simulink model "Emergency_Power_R2020a"  (R2020a)
settings: Solver=VariableStepAuto  StartTime=0.0  StopTime=10.0  RelTol=1e-3
undefined symbols (not defined in the file or in its folder): Ion, Lithium
libraries: electricdrivelib x29, powerlib x13
settings Model: Creator=YXL1108  LastModifiedBy=YXL1108

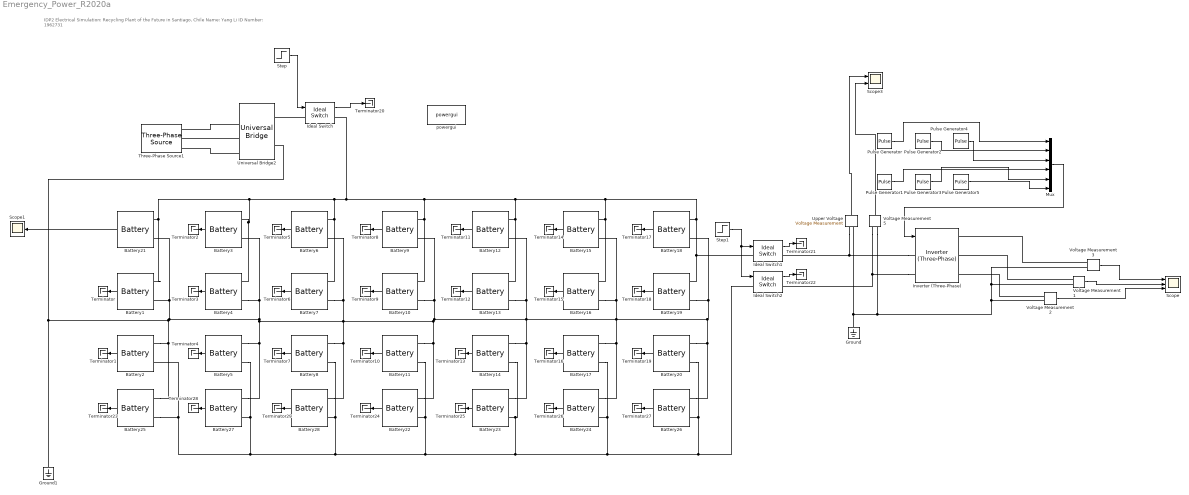
== system Emergency_Power_R2020a ==
  note: IDP2 Electrical Simulation: Recycling Plant of the Future in Santiago, Chile
      | Name: Yang Li
      | ID Number: 1962731
  Battery{1..28} (28 alike) : electricdrivelib/Extra Sources/Battery  BatType=Lithium-Ion  ShowTempParam=off  ThermalPreset=no  ShowAgeParam=off  NomV=Battery_nominal_v  NomQ=Rated_capacity  SOC=100  Batt_Tr=30  PresetModel=on  MaxQ=1000000  MinV=285  FullV=442.3151  Dis_rate=434782.6087  R=3.8e-06  Normal_OP=904347.8261  expZone="[410.546624      49130.4348]"  current=[6.5 13 32.5]  Units=Time  Tci=20  NomT=20  T2=-30  MaxQ2=4.8  FullV2=7.1  Normal_OP2=5.655  expZone2="[6.58           1]"  Rca=0.6  ti=2000  Dp=0  Neq0=0  Tsim=1e6  Ta1=25  Qeol=5.4*0.9  Reol=0.013333*1.2  Char_age=[2.3478, 3]  Dis_age=[2.3478, 10]  N1=1500  N2=10500  N3=1000  N4=1400  Ta2=45  N5=950
  Ground : powerlib/Elements/Ground  LConnTagsString=a
  Ground1 : powerlib/Elements/Ground  LConnTagsString=a
  Ideal Switch : powerlib/Power Electronics/Ideal Switch  Ron=0.001  Lon=0  IC=0  Rs=1e-5  Cs=inf  Measurements=on
  Ideal Switch1 : powerlib/Power Electronics/Ideal Switch  Ron=0.001  Lon=0  IC=0  Rs=1e-5  Cs=inf  Measurements=on
  Ideal Switch2 : powerlib/Power Electronics/Ideal Switch  Ron=0.001  Lon=0  IC=0  Rs=1e-5  Cs=inf  Measurements=on
  Inverter (Three-Phase) : electricdrivelib/Fundamental Drive Blocks/Inverter (Three-Phase)  LabelModeActiveChoice=Detailed  detailLevel=Detailed  driveType=Field-oriented control  Ts=2e-6  SnubberResistance=10e3  SnubberCapacitance=inf  Device=MOSFET / Diodes  Ron=1e-3  ForwardVoltages=[1.2,1.2]  GTOparameters=[1e-6,2e-6]  IGBTparameters=[1e-6,2e-6]  Measurements=All voltages and currents  converterType=Inverter  SourceFrequency=60  ReferenceFrame=Rotor  dqInductances=[8.5e-3,8.5e-3]  Inductance=8.5e-3  Ls=0  Resistance=0.2  Flux=0.175  Stator_sm=[2.01e-3,4.289e-4,4.477e-3,1.354e-3]  Stator_im=[14.85e-3,0.3027e-3]  Rotor=[9.295e-3,0.3027e-3]  Lm=10.46e-3  p=4
      settings: AttributesFormatString=%<BlockChoice>  SourceProductBaseCode=PS
  Mux : Mux  Inputs=6
  Pulse Generator : DiscretePulseGenerator  PulseType=Time based  Period=0.02  PulseWidth=33.33
  Pulse Generator1 : DiscretePulseGenerator  PulseType=Time based  Period=0.02  PulseWidth=33.33  PhaseDelay=9.99e-3
  Pulse Generator2 : DiscretePulseGenerator  PulseType=Time based  Period=0.02  PulseWidth=33.33  PhaseDelay=6.66e-3
  Pulse Generator3 : DiscretePulseGenerator  PulseType=Time based  Period=0.02  PulseWidth=33.33  PhaseDelay=0.01665
  Pulse Generator4 : DiscretePulseGenerator  PulseType=Time based  Period=0.02  PulseWidth=33.33  PhaseDelay=0.01332
  Pulse Generator5 : DiscretePulseGenerator  PulseType=Time based  Period=0.02  PulseWidth=33.33  PhaseDelay=3.33e-3
  Scope : Scope  NumInputPorts=3
  Scope1 : Scope
  Scope3 : Scope  NumInputPorts=2
  Step : Step  Time=5  SampleTime=0
  Step1 : Step  Time=5  Before=1  After=0  SampleTime=0
  Terminator{,1..29} (30 alike) : Terminator
  Three-Phase Source1 : powerlib/Electrical Sources/Three-Phase Source  InternalConnection=Yg  VoltagePhases=off  Voltage=25e3  PhaseAngle=0  Voltage_phases=[25e3 25e3 25e3]/sqrt(3)  PhaseAngles_phases=[0 -120 +120]  Frequency=60  NonIdealSource=on  SpecifyImpedance=off  Resistance=0.8929  Inductance=16.58e-3  ShortCircuitLevel=100e6  BaseVoltage=25e3  XRratio=7  BusType=swing  Pref=10e3  Qref=0  Prefabc=[10e3, 10e3, 10e3]  Qrefabc=[0, 0, 0]  Qmin=-inf  Qmax=inf
  Universal Bridge2 : powerlib/Power Electronics/Universal Bridge  Arms=3  SnubberResistance=1e5  SnubberCapacitance=inf  Device=Thyristors  Ron=1e-3  Lon=0  ForwardVoltages="[  0  0  ]"  ForwardVoltage=0  GTOparameters=[ 10e-6 , 20e-6 ]  IGBTparameters=[ 1e-6 , 2e-6 ]  Measurements=None  Measurements_2=None  converterType=Rectifier
  Upper Voltage : powerlib/Measurements/Voltage Measurement  PhasorSimulation=off  OutputType=Complex  PSBequivalent=0
  Voltage Measurement{1..3,5} (4 alike) : powerlib/Measurements/Voltage Measurement  PhasorSimulation=off  OutputType=Complex  PSBequivalent=0
  powergui : powerlib/powergui  Priority=1  SimulationMode=Continuous  SampleTime=50e-6  frequency=60  Iterations=50  frequencyindice=60  Pbase=100e6  ErrMax=1e-4  UnitsV=kV  UnitsW=MW  buscounter=0  FunctionMessages=off  echomessages=off  EnableUseOfTLC=off  CurrentSourceSwitches=off  DisableSnubberDevices=off  DisableRonSwitches=off  DisableVfSwitches=off  DisplayEquations=off  AutomaticDiscreteSolvers=off  SolverType=Tustin/Backward Euler (TBE)  Interpol=off  ExternalGateDelay=off  methode=off  Ts=100  x0status=blocks  SPID=on  SwTol=0  HookPort=off  NonlinearTolerance=1e-4  nMaxIteration=100  ContinueOnMaxIteration=off  RestoreLinks=warning  ResistiveCurrentMeasurement=off  Frange=[0:2:500]  Ylog=off  Xlog=on  ShowGrid=off  save=off  variable=ZData  structure=0  ZoomFFT=off  StartTime=0.0  cycles=1  DisplayStyle=1  fundamental=60  FreqAxis=off  MaxFrequency=1000  frequencyindicesteady=1  RmsSteady=1  display=off
  wires:
  Voltage Measurement3/1 -> Scope/1
  Voltage Measurement1/1 -> Scope/2
  Voltage Measurement2/1 -> Scope/3
  Step/1 -> Ideal Switch/1
  Battery21/1 -> Scope1/1
  Battery1/1 -> Terminator/1
  Battery2/1 -> Terminator1/1
  Battery3/1 -> Terminator2/1
  Battery4/1 -> Terminator3/1
  Battery5/1 -> Terminator4/1
  Battery6/1 -> Terminator5/1
  Battery7/1 -> Terminator6/1
  Battery8/1 -> Terminator7/1
  Battery9/1 -> Terminator8/1
  Battery10/1 -> Terminator9/1
  Battery12/1 -> Terminator11/1
  Battery13/1 -> Terminator12/1
  Battery14/1 -> Terminator13/1
  Battery11/1 -> Terminator10/1
  Battery15/1 -> Terminator14/1
  Battery16/1 -> Terminator15/1
  Battery17/1 -> Terminator16/1
  Battery18/1 -> Terminator17/1
  Battery19/1 -> Terminator18/1
  Battery20/1 -> Terminator19/1
  Pulse Generator/1 -> Mux/1
  Pulse Generator2/1 -> Mux/2
  Pulse Generator4/1 -> Mux/3
  Pulse Generator1/1 -> Mux/4
  Pulse Generator3/1 -> Mux/5
  Pulse Generator5/1 -> Mux/6
  Mux/1 -> Inverter (Three-Phase)/1
  Upper Voltage/1 -> Scope3/1
  Voltage Measurement5/1 -> Scope3/2
  Ideal Switch/1 -> Terminator20/1
  Step1/1 -> Ideal Switch1/1, Ideal Switch2/1
  Ideal Switch1/1 -> Terminator21/1
  Ideal Switch2/1 -> Terminator22/1
  Battery26/1 -> Terminator27/1
  Battery24/1 -> Terminator26/1
  Battery22/1 -> Terminator24/1
  Battery23/1 -> Terminator25/1
  Battery28/1 -> Terminator29/1
  Battery27/1 -> Terminator28/1
  Battery25/1 -> Terminator23/1
  connections:
  Universal Bridge2/LConn2 -- Three-Phase Source1/RConn2
  Universal Bridge2/LConn1 -- Three-Phase Source1/RConn1
  Universal Bridge2/LConn3 -- Three-Phase Source1/RConn3
  Battery1/LConn1 -- Battery21/LConn1 -- Ideal Switch/RConn1 -- Ideal Switch1/LConn1 -- Battery19/LConn1 -- Battery18/LConn1 -- Battery16/LConn1 -- Battery15/LConn1 -- Battery13/LConn1 -- Battery12/LConn1 -- Battery10/LConn1 -- Battery9/LConn1 -- Battery7/LConn1 -- Battery6/LConn1 -- Battery4/LConn1 -- Battery3/LConn1
  Ideal Switch/LConn1 -- Universal Bridge2/RConn1
  Inverter (Three-Phase)/LConn1 -- Ideal Switch1/RConn1 -- Upper Voltage/LConn1
  Voltage Measurement1/LConn1 -- Inverter (Three-Phase)/RConn2
  Voltage Measurement3/LConn1 -- Inverter (Three-Phase)/RConn1
  Voltage Measurement2/LConn1 -- Inverter (Three-Phase)/RConn3
  Inverter (Three-Phase)/LConn2 -- Ideal Switch2/RConn1 -- Voltage Measurement5/LConn1
  Voltage Measurement1/LConn2 -- Upper Voltage/LConn2 -- Ground/LConn1 -- Voltage Measurement5/LConn2 -- Voltage Measurement2/LConn2 -- Voltage Measurement3/LConn2
  Ground1/LConn1 -- Battery25/LConn1 -- Battery2/LConn1 -- Battery27/LConn1 -- Battery5/LConn1 -- Battery28/LConn1 -- Battery8/LConn1 -- Battery22/LConn1 -- Battery11/LConn1 -- Battery10/LConn2 -- Battery9/LConn2 -- Battery23/LConn1 -- Battery14/LConn1 -- Battery24/LConn1 -- Battery17/LConn1 -- Battery26/LConn1 -- Battery20/LConn1 -- Battery18/LConn2 -- Battery19/LConn2 -- Battery16/LConn2 -- Battery15/LConn2 -- Battery13/LConn2 -- Battery12/LConn2 -- Battery7/LConn2 -- Battery6/LConn2 -- Battery4/LConn2 -- Battery3/LConn2 -- Battery1/LConn2 -- Battery21/LConn2 -- Universal Bridge2/RConn2
  Battery20/LConn2 -- Battery23/LConn2 -- Battery14/LConn2 -- Battery11/LConn2 -- Battery22/LConn2 -- Battery28/LConn2 -- Battery8/LConn2 -- Battery27/LConn2 -- Battery5/LConn2 -- Battery25/LConn2 -- Battery2/LConn2 -- Battery24/LConn2 -- Battery17/LConn2 -- Ideal Switch2/LConn1 -- Battery26/LConn2
